simulink model "PD_controller"  (R2020a)
settings: Solver=VariableStepAuto  StartTime=0.0  StopTime=10.0  RelTol=1e-3
values from neighbouring files (symbols this model uses):
  Kpd = -(alpha_1 + alpha_2) /K_1    (= 9.70825688073)    [lab_1_init.m]
  Kpp = (alpha_1*alpha_2 + beta*beta)/K_1    (= 12.6020642202)    [lab_1_init.m]
settings Model: Creator=olav_  LastModifiedBy=olav_

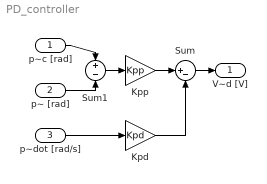
== system PD_controller ==
  p~c [rad] : Inport
  p~ [rad] : Inport  Port=2
  p~dot [rad/s] : Inport  Port=3
  Kpd : Gain  Gain=Kpd
  Kpp : Gain  Gain=Kpp
  Sum : Sum  Inputs=|+-
  Sum1 : Sum  Inputs=+|-
  V~d [V] : Outport  InitialOutput=0
  wires:
  Kpd/1 -> Sum/2
  Sum1/1 -> Kpp/1
  p~c [rad]/1 -> Sum1/1
  p~ [rad]/1 -> Sum1/2
  Kpp/1 -> Sum/1
  p~dot [rad/s]/1 -> Kpd/1
  Sum/1 -> V~d [V]/1
